simulink model "Project_microgrid__2016a"  (R2016a)
settings: Solver=VariableStepAuto  SolverMode=SingleTasking  StartTime=0.0  StopTime=0.3  RelTol=1e-3
undefined symbols (not defined in the file): D1, D11, Delta, DiscIntNeverNeededParam, find_system, Hydride, Metal, Nickel
libraries: powerlib x77, powerlib_meascontrol x31, sps_avr x7, simulink_extras x4, simulink x3, electricdrivelib x1, spsDieselMotorModel x1, re_lib x1
(part 2 of 5)

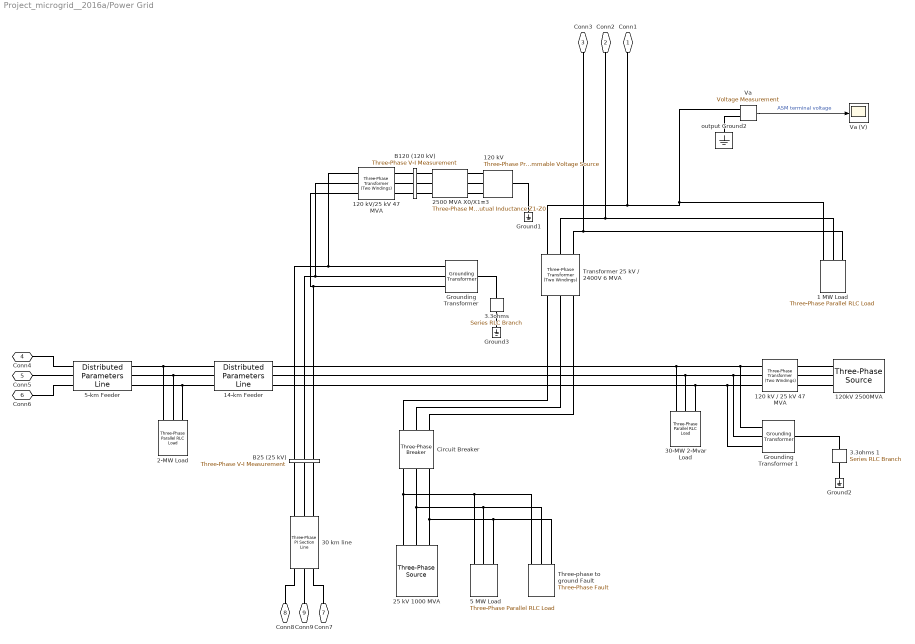
== system Project_microgrid__2016a/Power Grid ==
  1 MW Load : powerlib/Elements/Three-Phase Parallel RLC Load  LConnTagsString=A|B|C  Configuration=Y (grounded)  NominalVoltage=2400  Vabc=[1e3 1e3 1e3]  Vabcp=[1e3 1e3 1e3]  NominalFrequency=60  UnbalancedPower=off  ActivePower=1e+006  InductivePower=0  CapacitivePower=0  Pabc=[10e3 9e3 11e3]  QLabc=[100 90 110]  QCabc=[100 90 110]  Pabcp=[10e3 9e3 11e3]  QLabcp=[100 90 110]  QCabcp=[100 90 110]  Measurements=None  LoadType=constant Z
  120 kV : powerlib/Electrical Sources/Three-Phase Programmable Voltage Source  PositiveSequence=[120e3 0 60]  VariationEntity=Amplitude  VariationType=Table of time-amplitude pairs  VariationTypeAlt=Step  VariationStep=-0.2  VariationRate=10  VariationMagnitude=0.3  VariationFrequency=2  VariationTiming=[0.05 0.05+5/60]  VariationPhaseA=off  Amplitudes=[1 0.75 1.0]  TimeValues=[0 0.03 0.13]  HarmonicGeneration=off  HarmonicA=[1 -0.1 0 2]  HarmonicB=[2 0.15 35 2]*0  Timing="[0.1  2]"  BusType=swing  Pref=0  Qref=0  Qmin=-inf  Qmax=inf
  120 kV / 25 kV 47 MVA : powerlib/Elements/Three-Phase Transformer (Two Windings)  Winding1Connection=Yg  Winding2Connection=Delta (D1)  CoreType=Three single-phase transformers  SetSaturation=off  Hysteresis=off  DataFile='basic_model'  SetInitialFlux=off  Measurements=None  UNITS=pu  NominalPower=[47e6 50 ]  Winding1="[ 120e3  0.08/30   0.08 ]"  Winding2="[ 25e3  0.08/30  0.08]"  Rm=500  Lm=500  L0=0.5  Saturation="[ 0,0  ;  0.005,1.2  ;  1.0,1.4 ]"  InitialFluxes=[ 0.8 , -0.8 , 0.7 ]  BreakLoop=off  DiscreteSolver=Trapezoidal iterative  DataType=off  TransfoNumber=0
  120 kV/25 kV 47 MVA : powerlib/Elements/Three-Phase Transformer (Two Windings)  Winding1Connection=Yg  Winding2Connection=Delta (D1)  CoreType=Three single-phase transformers  SetSaturation=off  Hysteresis=off  DataFile='basic_model'  SetInitialFlux=off  Measurements=None  UNITS=pu  NominalPower=[47e6 60 ]  Winding1="[ 120e3  0.08/30   0.08 ]"  Winding2="[ 25e3  0.08/30  0.08]"  Rm=500  Lm=500  L0=0.5  Saturation="[ 0,0  ;  0.005,1.2  ;  1.0,1.4 ]"  InitialFluxes=[ 0.8 , -0.8 , 0.7 ]  BreakLoop=off  DiscreteSolver=Trapezoidal iterative  DataType=off  TransfoNumber=0
  120kV 2500MVA : powerlib/Electrical Sources/Three-Phase Source  InternalConnection=Yg  VoltagePhases=off  Voltage=150e3  PhaseAngle=0  Voltage_phases=[25e3 25e3 25e3]/sqrt(3)  PhaseAngles_phases=[0 -120 +120]  Frequency=50  NonIdealSource=on  SpecifyImpedance=on  Resistance=0.8929  Inductance=16.58e-3  ShortCircuitLevel=2500e6  BaseVoltage=120e3  XRratio=7  BusType=swing  Pref=0  Qref=0  Prefabc=[10e3, 10e3, 10e3]  Qrefabc=[0, 0, 0]  Qmin=-inf  Qmax=inf
  14-km Feeder : powerlib/Elements/Distributed Parameters Line  Phases=3  Frequency=50  Resistance=[0.1153 0.413]  Inductance=[1.05e-3 3.32e-3]  Capacitance=[11.33e-009 5.01e-009]  Length=14  x1=[-6e-05 5.24389383888345e-09 0 0;-5.6e-05 5.24712174909757e-09 0 0;-5.2e-05 5.25034137339023e-09 -4592.41120839546 -30084.6016905143;-4.8e-05 5.25355270667721e-09 -4554.60216686054 -30090.348929275;-4.4e-05 5.25675574388738e-09 -4516.7859329871 -30096.0486512675;-4e-05 5.2599504799627e-09 -4478.96256649216 -30101.7008474912;-3.6e-05 5.26313690985824e-09 -4441.13212710396 -30107.3055090205;-3.2e-05 5.26631502854221e-09 -4403.29467456193 -30112.8626270048;-2.8e-05 5.26948483099591e-09 -4365.45026861658 -30118.3721926688;-2.4e-05 5.27264631221381e-09 -4327.59896902939 -30123.834197312;-2e-05 5.27579946720347e-09 -4289.74083557272 -30129.2486323092;-1.6e-05 5.27894429098565e-09 -4251.87592802974 -30134.6154891103;-1.2e-05 5.28208077859424e-09 -4214.0043061943 -30139.9347592403;-8e-06 5.28520892507629e-09 -4176.12602987087 -30145.2064342993;-4e-06 5.28832872549204e-09 -4138.24115887441 -30150.4305059626]  x2=[-6e-05 5.41313383180429e-09 0 0;-5.6e-05 5.41611613444594e-09 0 0;-5.2e-05 5.41908988430093e-09 -4166.95541576399 -30299.6062453431;-4.8e-05 5.4220550766733e-09 -4128.87652753458 -30304.8186709667;-4.4e-05 5.42501170688062e-09 -4090.79111924556 -30309.9832411452;-4e-05 5.42795977025396e-09 -4052.69925103899 -30315.0999477229;-3.6e-05 5.43089926213792e-09 -4014.60098306712 -30320.1687826199;-3.2e-05 5.43383017789066e-09 -3976.49637549232 -30325.1897378317;-2.8e-05 5.43675251288384e-09 -3938.38548848696 -30330.1628054297;-2.4e-05 5.43966626250271e-09 -3900.26838223334 -30335.0879775607;-2e-05 5.44257142214605e-09 -3862.14511692358 -30339.9652464471;-1.6e-05 5.44546798722623e-09 -3824.01575275951 -30344.7946043871;-1.2e-05 5.44835595316917e-09 -3785.88034995259 -30349.5760437545;-8e-06 5.45123531541438e-09 -3747.73896872385 -30354.3095569987;-4e-06 5.45410606941495e-09 -3709.59166930372 -30358.9951366449]  x3=[-6e-05 2.19439041380111e-11 0 0;-5.6e-05 2.1954853930582e-11 0 0;-5.2e-05 2.19657690534419e-11 -28.5335833203508 -194.664312913599;-4.8e-05 2.19766494893542e-11 -28.2889384653752 -194.700015561698;-4.4e-05 2.19874952211371e-11 -28.0442489383045 -194.735410751896;-4e-05 2.1998306231664e-11 -27.7995151255367 -194.770498428299;-3.6e-05 2.20090825038626e-11 -27.55473741354 -194.8052785355;-3.2e-05 2.20198240207157e-11 -27.3099161888519 -194.839751018577;-2.8e-05 2.20305307652612e-11 -27.0650518380783 -194.873915823091;-2.4e-05 2.20412027205914e-11 -26.8201447478936 -194.907772895093;-2e-05 2.2051839869854e-11 -26.5751953050395 -194.941322181117;-1.6e-05 2.20624421962515e-11 -26.3302038963246 -194.974563628185;-1.2e-05 2.20730096830412e-11 -26.0851709086238 -195.007497183803;-8e-06 2.20835423135359e-11 -25.8400967288776 -195.040122795965;-4e-06 2.20940400711028e-11 -25.5949817440916 -195.072440413152]  x4=[-6e-05 -8.98993550684834e-12 0 0;-5.6e-05 -8.99242296522254e-12 0 0;-5.2e-05 -8.99489622333346e-12 -1.62633633076446 -2.68614935355567;-4.8e-05 -8.99735527727546e-12 -1.62295953271912 -2.6881909466271;-4.4e-05 -8.99980012316538e-12 -1.61958017179915 -2.69022829467809;-4e-05 -9.00223075714246e-12 -1.61619825334102 -2.6922613944914;-3.6e-05 -9.0046471753684e-12 -1.61281378268524 -2.69429024285649;-3.2e-05 -9.00704937402735e-12 -1.60942676517636 -2.69631483656952;-2.8e-05 -9.00943734932591e-12 -1.60603720616294 -2.69833517243338;-2.4e-05 -9.01181109749315e-12 -1.60264511099754 -2.7003512472577;-2e-05 -9.01417061478057e-12 -1.59925048503676 -2.70236305785881;-1.6e-05 -9.0165158974622e-12 -1.59585333364118 -2.70437060105978;-1.2e-05 -9.0188469418345e-12 -1.59245366217535 -2.70637387369045;-8e-06 -9.02116374421644e-12 -1.58905147600782 -2.70837287258735;-4e-06 -9.02346630094948e-12 -1.58564678051112 -2.71036759459381]  x5=5.70973484498186e-05  V1=ones(3,3)  V2=ones(3,3)  I1=ones(3,3)  I2=ones(3,3)  nHarmo=1  Measurements=None
  2-MW Load : powerlib/Elements/Three-Phase Parallel RLC Load  LConnTagsString=A|B|C  Configuration=Y (grounded)  NominalVoltage=25e3  Vabc=[1e3 1e3 1e3]  Vabcp=[1e3 1e3 1e3]  NominalFrequency=50  UnbalancedPower=off  ActivePower=2e6  InductivePower=0  CapacitivePower=0  Pabc=[10e3 9e3 11e3]  QLabc=[100 90 110]  QCabc=[100 90 110]  Pabcp=[10e3 9e3 11e3]  QLabcp=[100 90 110]  QCabcp=[100 90 110]  Measurements=None  LoadType=constant Z
  25 kV 1000 MVA : powerlib/Electrical Sources/Three-Phase Source  InternalConnection=Yg  VoltagePhases=off  Voltage=(25000)*1  PhaseAngle=2.1395e-05  Voltage_phases=[25e3 25e3 25e3]/sqrt(3)  PhaseAngles_phases=[0 -120 +120]  Frequency=60  NonIdealSource=on  SpecifyImpedance=on  Resistance=25^2/1000/10  Inductance=25^2/1000/377  ShortCircuitLevel=1000e6  BaseVoltage=25e3  XRratio=10  BusType=swing  Pref=0  Qref=0  Prefabc=[10e3, 10e3, 10e3]  Qrefabc=[0, 0, 0]  Qmin=-Inf  Qmax=Inf
  2500 MVA X0/X1=3 : powerlib/Elements/Three-Phase Mutual Inductance Z1-Z0  LConnTagsString=a|b|c  RConnTagsString=A|B|C  PositiveSequence="[0.1  1.0/(2*pi*60)] *120e3^2/2500e6"  ZeroSequence="[0.3  3.0/(2*pi*60)] *120e3^2/2500e6"
  "3.3ohms " : powerlib/Elements/Series RLC Branch  LConnTagsString=__new0  RConnTagsString=__new0  BranchType=R  Resistance=3.3  Inductance=[]  SetiL0=off  InitialCurrent=0  Capacitance=[]  Setx0=off  InitialVoltage=0  Measurements=None
  3.3ohms 1 : powerlib/Elements/Series RLC Branch  LConnTagsString=__new0  RConnTagsString=__new0  BranchType=R  Resistance=3.3  Inductance=[]  SetiL0=off  InitialCurrent=0  Capacitance=[]  Setx0=off  InitialVoltage=0  Measurements=None
  30 km line : powerlib/Elements/Three-Phase PI Section Line  LConnTagsString=a|b|c  RConnTagsString=A|B|C  Frequency=60  Resistances=[0.1153 0.413]  Inductances=[1.05e-3 3.32e-3]  Capacitances=[11.33e-009 5.01e-009]  Length=30
  30-MW 2-Mvar Load : powerlib/Elements/Three-Phase Parallel RLC Load  LConnTagsString=A|B|C  Configuration=Y (grounded)  NominalVoltage=25e3  Vabc=[1e3 1e3 1e3]  Vabcp=[1e3 1e3 1e3]  NominalFrequency=50  UnbalancedPower=off  ActivePower=30e6  InductivePower=2e6  CapacitivePower=0  Pabc=[10e3 9e3 11e3]  QLabc=[100 90 110]  QCabc=[100 90 110]  Pabcp=[10e3 9e3 11e3]  QLabcp=[100 90 110]  QCabcp=[100 90 110]  Measurements=None  LoadType=constant Z
  5 MW Load : powerlib/Elements/Three-Phase Parallel RLC Load  LConnTagsString=A|B|C  Configuration=Y (grounded)  NominalVoltage=25e3  Vabc=[1e3 1e3 1e3]  Vabcp=[1e3 1e3 1e3]  NominalFrequency=60  UnbalancedPower=off  ActivePower=5e+006  InductivePower=0  CapacitivePower=0  Pabc=[10e3 9e3 11e3]  QLabc=[100 90 110]  QCabc=[100 90 110]  Pabcp=[10e3 9e3 11e3]  QLabcp=[100 90 110]  QCabcp=[100 90 110]  Measurements=None  LoadType=constant Z
  5-km Feeder : powerlib/Elements/Distributed Parameters Line  Phases=3  Frequency=50  Resistance=[0.1153 0.413]  Inductance=[1.05e-3 3.32e-3]  Capacitance=[11.33e-009 5.01e-009]  Length=5  x1=[-2.4e-05 5.33826007366157e-09 -4328.38679732203 -30125.1982220609;-2e-05 5.34139179699889e-09 -4290.52694915972 -30130.6136459951;-1.6e-05 5.34451508554948e-09 -4252.66032566971 -30135.9814895777;-1.2e-05 5.34762993438124e-09 -4214.78698664858 -30141.301744332;-8e-06 5.35073633857541e-09 -4176.90699190349 -30146.5744018567;-4e-06 5.35383429322654e-09 -4139.02040125213 -30151.7994538255]  x2=[-2.4e-05 5.27264631221381e-09 -4327.59896902939 -30123.834197312;-2e-05 5.27579946720347e-09 -4289.74083557272 -30129.2486323092;-1.6e-05 5.27894429098565e-09 -4251.87592802974 -30134.6154891103;-1.2e-05 5.28208077859424e-09 -4214.0043061943 -30139.9347592403;-8e-06 5.28520892507629e-09 -4176.12602987087 -30145.2064342993;-4e-06 5.28832872549204e-09 -4138.24115887441 -30150.4305059626]  x3=[-2.4e-05 2.33940631713485e-13 -13.5809735435642 -98.9468276004231;-2e-05 2.2688527897437e-13 -13.4566226025095 -98.9638158253433;-1.6e-05 2.19829567952431e-13 -13.332250411611 -98.9806477728902;-1.2e-05 2.12773509789599e-13 -13.2078571672692 -98.9973234164837;-8e-06 2.05717115628352e-13 -13.0834430659182 -99.0138427297907;-4e-06 1.98660396611699e-13 -12.9590083040247 -99.030205686725]  x4=[-2.4e-05 1.33449662502356e-11 -15.3482236981344 -98.6065510111038;-2e-05 1.33597788176704e-11 -15.2242989657759 -98.6257602961521;-1.6e-05 1.33745702881909e-11 -15.1003501921712 -98.6448138376629;-1.2e-05 1.33893406384393e-11 -14.9763775730525 -98.6637116055479;-8e-06 1.34040898450913e-11 -14.8523813041894 -98.6824535699651;-4e-06 1.34188178848558e-11 -14.7283615813888 -98.7010397013183]  x5=2.03919101606495e-05  V1=ones(3,3)  V2=ones(3,3)  I1=ones(3,3)  I2=ones(3,3)  nHarmo=1  Measurements=None
  B120 (120 kV) : powerlib/Measurements/Three-Phase V-I Measurement  VoltageMeasurement=no  SetLabelV=off  LabelV=Vabc_B120  Vpu=off  VpuLL=off  CurrentMeasurement=no  SetLabelI=on  LabelI=Iabc_B120  Ipu=off  Pbase=100e6  Vbase=120e3  OutputType=Complex  PhasorSimulation=off  PSBequivalent=0
  B25 (25 kV) : powerlib/Measurements/Three-Phase V-I Measurement  VoltageMeasurement=phase-to-ground  SetLabelV=on  LabelV=Vabc_B25  Vpu=off  VpuLL=off  CurrentMeasurement=yes  SetLabelI=on  LabelI=Iabc_B25  Ipu=off  Pbase=10e6  Vbase=25e3  OutputType=Complex  PhasorSimulation=off  PSBequivalent=0
  Circuit Breaker : powerlib/Elements/Three-Phase Breaker  InitialState=closed  SwitchA=on  SwitchB=on  SwitchC=on  SwitchTimes=[0.2]  External=off  BreakerResistance=0.01  SnubberResistance=1e5  SnubberCapacitance=inf  Measurements=None
      settings: AttributesFormatString=\n
  Ground1 : powerlib/Elements/Ground  LConnTagsString=a
  Ground2 : powerlib/Elements/Ground  LConnTagsString=a
  Ground3 : powerlib/Elements/Ground  LConnTagsString=a
  "Grounding Transformer " : powerlib/Elements/Grounding Transformer   UNITS=pu  NominalPower="[100e6   60]"  NominalVoltage=25e3  ZeroSequenceImpedance_pu=[0.025 0.75]  MagnetizationBranch_pu=[500 500]  ZeroSequenceImpedance_SI=[0.052083 589.05]  MagnetizationBranch_SI=[1041.7 3.927e+005]  Measurements=None
  Grounding Transformer 1 : powerlib/Elements/Grounding Transformer   UNITS=pu  NominalPower="[150e6   50]"  NominalVoltage=25e3  ZeroSequenceImpedance_pu=[0.025 0.75]  MagnetizationBranch_pu=[500 500]  ZeroSequenceImpedance_SI=[0.052083 589.05]  MagnetizationBranch_SI=[1041.7 3.927e+005]  Measurements=None
  Three-phase to ground Fault : powerlib/Elements/Three-Phase Fault  InitialStates=0  FaultA=on  FaultB=on  FaultC=on  GroundFault=on  SwitchTimes=[ 0.1 0.4]  External=off  SwitchStatus=NaN  FaultResistance=0.01  GroundResistance=0.001  SnubberResistance=inf  SnubberCapacitance=inf  Measurements=None
  Transformer 25 kV / 2400V 6 MVA : powerlib/Elements/Three-Phase Transformer (Two Windings)  Winding1Connection=Yg  Winding2Connection=Delta (D1)  CoreType=Three single-phase transformers  SetSaturation=off  Hysteresis=off  DataFile='hysteresis'  SetInitialFlux=off  Measurements=None  UNITS=pu  NominalPower=[ 6e6 , 60 ]  Winding1=[ 25e3 , 0.0015 , 0.03]  Winding2=[ 2.4e3 , 0.0015 , 0.03 ]  Rm=200  Lm=200  L0=0.5  Saturation="[ 0,0  ;  0.005,1.2  ;  1.0,1.4 ]"  InitialFluxes=[ 0.8 , -0.8 , 0.7 ]  BreakLoop=off  DiscreteSolver=Trapezoidal iterative  DataType=off  TransfoNumber=0
  Va : powerlib/Measurements/Voltage Measurement  Tag=PoWeRsYsTeMmEaSuReMeNt  PhasorSimulation=off  OutputType=Magnitude  PSBequivalent=0
  Va (V) : Scope
  output Ground2 : powerlib/Elements/Ground  LConnTagsString=a
  Conn1 : PMIOPort  Side=Left
  Conn2 : PMIOPort  Port=2  Side=Left
  Conn3 : PMIOPort  Port=3  Side=Left
  Conn4 : PMIOPort  Port=4  Side=Left
  Conn5 : PMIOPort  Port=5  Side=Left
  Conn6 : PMIOPort  Port=6  Side=Left
  Conn7 : PMIOPort  Port=7  Side=Left
  Conn8 : PMIOPort  Port=8  Side=Left
  Conn9 : PMIOPort  Port=9  Side=Left
  wires:
  Va/1 -> Va (V)/1  "ASM terminal voltage"
  connections:
  B120 (120 kV)/RConn1 -- 120 kV/25 kV 47 MVA/LConn1
  "3.3ohms "/RConn1 -- Ground3/LConn1
  Circuit Breaker/LConn1 -- 25 kV 1000 MVA/RConn1 -- 5 MW Load/LConn1 -- Three-phase to ground Fault/LConn1
  "Grounding Transformer "/LConn3 -- 120 kV/25 kV 47 MVA/RConn3 -- B25 (25 kV)/LConn3
  B120 (120 kV)/RConn3 -- 120 kV/25 kV 47 MVA/LConn3
  25 kV 1000 MVA/RConn3 -- Circuit Breaker/LConn3 -- 5 MW Load/LConn3 -- Three-phase to ground Fault/LConn3
  Conn6/RConn1 -- 5-km Feeder/LConn3
  Transformer 25 kV / 2400V 6 MVA/RConn3 -- Conn3/RConn1 -- 1 MW Load/LConn3
  2-MW Load/LConn3 -- 5-km Feeder/RConn3 -- 14-km Feeder/LConn3
  B120 (120 kV)/LConn3 -- 2500 MVA X0/X1=3/RConn3
  "3.3ohms "/LConn1 -- "Grounding Transformer "/RConn1
  120 kV/RConn1 -- 2500 MVA X0/X1=3/LConn1
  120 kV / 25 kV 47 MVA/LConn1 -- 120kV 2500MVA/RConn1
  120 kV / 25 kV 47 MVA/LConn2 -- 120kV 2500MVA/RConn2
  B25 (25 kV)/RConn3 -- 30 km line/LConn3
  B120 (120 kV)/LConn2 -- 2500 MVA X0/X1=3/RConn2
  2-MW Load/LConn2 -- 5-km Feeder/RConn2 -- 14-km Feeder/LConn2
  Transformer 25 kV / 2400V 6 MVA/RConn2 -- Conn2/RConn1 -- 1 MW Load/LConn2
  120 kV/RConn3 -- 2500 MVA X0/X1=3/LConn3
  30-MW 2-Mvar Load/LConn3 -- 14-km Feeder/RConn3 -- 120 kV / 25 kV 47 MVA/RConn3 -- Grounding Transformer 1/LConn3
  B25 (25 kV)/LConn2 -- "Grounding Transformer "/LConn2 -- 120 kV/25 kV 47 MVA/RConn2
  B120 (120 kV)/LConn1 -- 2500 MVA X0/X1=3/RConn1
  Grounding Transformer 1/RConn1 -- 3.3ohms 1/LConn1
  B25 (25 kV)/RConn1 -- 30 km line/LConn1
  120 kV/RConn2 -- 2500 MVA X0/X1=3/LConn2
  Conn9/RConn1 -- 30 km line/RConn2
  120 kV / 25 kV 47 MVA/LConn3 -- 120kV 2500MVA/RConn3
  Ground1/LConn1 -- 120 kV/LConn1
  B25 (25 kV)/RConn2 -- 30 km line/LConn2
  2-MW Load/LConn1 -- 5-km Feeder/RConn1 -- 14-km Feeder/LConn1
  30-MW 2-Mvar Load/LConn1 -- 120 kV / 25 kV 47 MVA/RConn1 -- Grounding Transformer 1/LConn1 -- 14-km Feeder/RConn1
  30-MW 2-Mvar Load/LConn2 -- 120 kV / 25 kV 47 MVA/RConn2 -- Grounding Transformer 1/LConn2 -- 14-km Feeder/RConn2
  B25 (25 kV)/LConn1 -- "Grounding Transformer "/LConn1 -- 120 kV/25 kV 47 MVA/RConn1
  B120 (120 kV)/RConn2 -- 120 kV/25 kV 47 MVA/LConn2
  3.3ohms 1/RConn1 -- Ground2/LConn1
  1 MW Load/LConn1 -- Va/LConn1 -- Transformer 25 kV / 2400V 6 MVA/RConn1 -- Conn1/RConn1
  Circuit Breaker/RConn2 -- Transformer 25 kV / 2400V 6 MVA/LConn2
  output Ground2/LConn1 -- Va/LConn2
  Three-phase to ground Fault/LConn2 -- 25 kV 1000 MVA/RConn2 -- Circuit Breaker/LConn2 -- 5 MW Load/LConn2
  Circuit Breaker/RConn3 -- Transformer 25 kV / 2400V 6 MVA/LConn3
  Circuit Breaker/RConn1 -- Transformer 25 kV / 2400V 6 MVA/LConn1
  Conn8/RConn1 -- 30 km line/RConn1
  Conn4/RConn1 -- 5-km Feeder/LConn1
  Conn5/RConn1 -- 5-km Feeder/LConn2
  Conn7/RConn1 -- 30 km line/RConn3

== system Project_microgrid__2016a/Relay G ==
  AC Time Overcurrent Relay2 : Subsystem  mask(AC Time Overcurrent Relay Block){tcpopup=Definite Minimum Time, k=0, alpha=0.02, B=0, PS=100%, TMS=0.1, TDS=5, CTpri=300, CTsec=5, Freq=60, RMSInit=0}
      mask prompts: tcpopup "Trip Characteristic"; PS "Plug Setting (PS) / Low-set (I >)"; TMS "Time Multiplier Setting (TMS)"; TDS "Time Delay Setting (TDS) in sec"; CTpri "Current Transformer Primary (A)"; CTsec "Current Transformer Secondary (A)"; Freq "Fundamental frequency (Hz):"; RMSInit "Initial RMS value:"
      mask help:
      | AC Time Overcurrent Relay Block developed by Dr Rodney Tan
      | Version 1.0 (Jun 2016)
      |
      | AC Time Overcurrent Relay (ANSI/IEEE C37.2 device number 51) that operates when the current exceeds a predetermined value.
      |
      | This relay operates with either a Definite Minimum Time (DMT) or Inverse Definite Minimum Time (IDMT) characteristic.
      |
      | This relay support both IEC 60255 Standard and IEEE Standard C37.112-1996 IDMT trip characteristic.
      mask Help:
      | <b><u>Block Setting</u></b>
      | <b>Trip Characteristic</b>
      | Relay operation mode selection of Definite Minimum Time (DMT), IEC 60255 Standard or IEEE Standard C37.112-1996 Inverse Definite Minimum Time (IDMT).
      | 
      | <b>Plug-Setting(PS) / Low-set (I >)</b>
      | Specify relay pick-up current based on current transformer rating ranging from 25% to 200% with 25% step interval.
      | 
      | <b>Time Multiplier Setting (TMS)</b>
      | Specify time delay multiplier ranging from 0.05 to 1.0 for IDMT relay operation. This setting will be disabled DMT relay operation mode.
      | 
      | <b>Plot Curve Button</b>
      | Plot current Inverse Definite Minimum Time trip curve.
      | 
      | <b>Time Delay Setting (TDS)</b>
      | Specify time delay ranging from 0.05sec to 99sec for Definite Minimum Time relay operation. This setting will be disabled in IDMT relay operation mode.
      | 
      | <b>Current Transformer Primary (A)</b>
      | Specify current transformer primary in Ampere.
      | 
      | <b>Current Transformer Secondary (A)</b>
      | Specify current transformer secondary in Ampere.
      | 
      | <b>Fundamental Frequency (Hz)</b>
      | Specify the RMS current measurement fundamental frequency, in hertz, of the input signal.
      | 
      | <b>Initial RMS Value</b>
      | Specify the RMS current measurement initial RMS value of the output signal.
      | 
      | <b><u>Block Input Output</u></b>
      | <b>I</b>
      | Current input to the AC time overcurrent relay
      | 
      | <b>trip</b>
      | Trip control signal output (1-0), commonly connected to circuit breaker
      | 
      | <b>OT</b>
      | Relay operating time output
      mask TypeOptions tcpopup: Definite Minimum Time | IEC Standard Inverse | IEC Very Inverse | IEC Long Time Inverse | IEC Extremely Inverse | IEC Ultra Inverse | IEEE Moderately Inverse | IEEE Very Inverse | IEEE Extremely Inverse
      mask Callback tcpopup:
      | switch(get_param(gcb,'tcpopup'))
      |     case 'IEC Standard Inverse'
      |         set_param(gcb,'k','0.14');
      |         set_param(gcb,'alpha','0.02');
      |         set_param(gcb,'B','0');
      |         set_param(gcb,'MaskEnables',{'on','off','off','off',...
      |                   'on','on','off','on','on','on','on'});
      |     case 'IEC Very Inverse'
      |         set_param(gcb,'k','13.5');
      |         set_param(gcb,'alpha','1');
      |         set_param(gcb,'B','0');
      |         set_param(gcb,'MaskEnables',{'on','off','off','off',...
      |                   'on','on','off','on','on','on','on'});
      |     case 'IEC Long Time Inverse'
      |         set_param(gcb,'k','120');
      |         set_param(gcb,'alpha','1');
      |         set_param(gcb,'B','0');
      |         set_param(gcb,'MaskEnables',{'on','off','off','off',...
      |                   'on','on','off','on','on','on','on'});
      |     case 'IEC Extremely Inverse'
      |         set_param(gcb,'k','80');
      |         set_param(gcb,'alpha','2');
      |         set_param(gcb,'B','0');
      |         set_param(gcb,'MaskEnables',{'on','off','off','off',...
      |                   'on','on','off','on','on','on','on'});
      |     case 'IEC Ultra Inverse'
      |         set_param(gcb,'k','315.2');
      |         set_param(gcb,'alpha','2.5');
      |         set_param(gcb,'B','0');
      |         set_param(gcb,'MaskEnables',{'on','off','off','off',...
      |                   'on','on','off','on','on','on','on'});
      |     case 'IEEE Moderately Inverse'
      |         set_param(gcb,'k','0.0515');
      |         set_param(gcb,'alpha','0.02');
      |         set_param(gcb,'B','0.114');
      |         set_param(gcb,'MaskEnables',{'on','off','off','off',...
      |                   'on','on','off','on','on','on','on'});
      |     case 'IEEE Very Inverse'
      |         set_param(gcb,'k','19.61');
      |         set_param(gcb,'alpha','2');
      |         set_param(gcb,'B','0.491');
      |         set_param(gcb,'MaskEnables',{'on','off','off','off',...
      |                   'on','on','off','on','on','on','on'});
      |     case 'IEEE Extremely Inverse'
      |         set_param(gcb,'k','28.2');
      |         set_param(gcb,'alpha','2');
      |         set_param(gcb,'B','0.1217');
      |         set_param(gcb,'MaskEnables',{'on','off','off','off',...
      |                   'on','on','off','on','on','on','on'});
      |     otherwise
      |         set_param(gcb,'k','0');
      |         set_param(gcb,'MaskEnables',{'on','off','off','off',...
      |                   'on','off','on','on','on','on','on'});
      | end
      mask TypeOptions PS: 25% | 50% | 75% | 100% | 125% | 150% | 175% | 200%
      mask TypeOptions TMS: 0.05 | 0.1 | 0.15 | 0.2 | 0.25 | 0.3 | 0.35 | 0.4 | 0.45 | 0.5 | 0.55 | 0.6 | 0.65 | 0.7 | 0.75 | 0.8 | 0.85 | 0.9 | 0.95 | 1.0
      mask Callback TDS:
      | TDS = str2double(get_param(gcb,'TDS'));
      | if (TDS > 99)||(TDS < 0.05)||isnan(TDS)
      |     msgbox('TDS must be in the range of 0.05-99 sec',...
      |     'Invalid Value !','error');
      |     set_param(gcb,'TDS','0.1');
      | end
      mask TypeOptions Freq: Irms/Freq
      mask TypeOptions RMSInit: Irms/RMSInit
      mask DialogControl plotbutton Prompt: Plot Curve
      mask DialogControl plotbutton Callback:
      | % Plotting IDMT Curve
      | TMS = str2num(get_param(gcb,'TMS'));
      | k = str2num(get_param(gcb,'k'));
      | alpha = str2num(get_param(gcb,'alpha'));
      | B = str2num(get_param(gcb,'B'));
      | I = 1:20;
      | td = ((k./((I.^alpha)-1))+B)*TMS;
      | loglog(td);
      | set(gcf, 'Position', [200 150 300 500]);
      | switch(get_param(gcb,'tcpopup'))
      |     case 'IEC Standard Inverse'
      |         title('IEC Standard Inverse');
      |         set(gca, 'YTick', (1:10));
      |         ylim([0.1 10]);
      |     case 'IEC Very Inverse'
      |         title('IEC Very Inverse');
      |         set(gca, 'YTick', (1:2:15));
      |         ylim([0.01 15]);
      |     case 'IEC Long Time Inverse'
      |         title('IEC Long Time Inverse');
      |         set(gca, 'YTick', (0:20:120));
      |         ylim([0.1 120]);
      |     case 'IEC Extremely Inverse'
      |         title('IEC Extremely Inverse');
      |         set(gca, 'YTick', (0:5:30));
      |         ylim([0.01 30]);
      |     case 'IEC Ultra Inverse'
      |         title('IEC Ultra Inverse');
      |         set(gca, 'YTick', (0:20:100));
      |         ylim([0.01 100]);
      |     case 'IEEE Moderately Inverse'
      |         title('IEEE Moderately Inverse');
      |         set(gca, 'YTick', (1:5));
      |         ylim([0.01 5]);
      |     case 'IEEE Very Inverse'
      |         title('IEEE Very Inverse');
      |         set(gca, 'YTick', (1:10));
      |         ylim([0.01 10]);
      |     case 'IEEE Extremely Inverse'
      |         title('IEEE Extremely Inverse');
      |         set(gca, 'YTick', (1:10));
      |         ylim([0.01 10]);
      | end
      | 
      | set(gca, 'XTick', [1:10 20]);
      | xlim([1 30]);
      | xlabel('Current (Multiples of Plug Setting)');
      | ylabel('Operating Time (sec)');
      | grid on;
      mask DialogControl RMS Prompt: RMS Current Measurement
      mask Display:
      | disp('(51)');
      | port_label('input', 1, 'I');
      | port_label('output', 1, 'trip');
      | port_label('output', 2, 'OT');
  Display : Display
  Output1 : Subsystem
  Three-Phase V-I Measurement : powerlib/Measurements/Three-Phase V-I Measurement  VoltageMeasurement=no  SetLabelV=off  LabelV=Vabc  Vpu=off  VpuLL=off  CurrentMeasurement=yes  SetLabelI=off  LabelI=Iabc  Ipu=off  Pbase=100e6  Vbase=500e3  OutputType=Complex  PhasorSimulation=off  PSBequivalent=0
  Three-Phase Breaker : powerlib/Elements/Three-Phase Breaker  InitialState=closed  SwitchA=on  SwitchB=on  SwitchC=on  SwitchTimes="[1/60  5/60]"  External=on  BreakerResistance=0.001  SnubberResistance=1e6  SnubberCapacitance=inf  Measurements=None
  A : PMIOPort  Side=Left
  a : PMIOPort  Port=2  Side=Right
  B : PMIOPort  Port=3  Side=Left
  b : PMIOPort  Port=4  Side=Right
  C : PMIOPort  Port=5  Side=Left
  c : PMIOPort  Port=6  Side=Right
  wires:
  Three-Phase V-I Measurement/1 -> Output1/1(Signal), AC Time Overcurrent Relay2/1(I)  "Iabc"
  AC Time Overcurrent Relay2/2(OT) -> Display/1
  AC Time Overcurrent Relay2/1(C.B) -> Three-Phase Breaker/1  "Relay C"
  connections:
  Three-Phase Breaker/RConn2 -- Three-Phase V-I Measurement/LConn2
  Three-Phase V-I Measurement/RConn2 -- b/RConn1
  Three-Phase V-I Measurement/LConn1 -- Three-Phase Breaker/RConn1
  Three-Phase Breaker/LConn2 -- B/RConn1
  Three-Phase V-I Measurement/RConn1 -- a/RConn1
  Three-Phase Breaker/RConn3 -- Three-Phase V-I Measurement/LConn3
  Three-Phase Breaker/LConn3 -- C/RConn1
  Three-Phase V-I Measurement/RConn3 -- c/RConn1
  Three-Phase Breaker/LConn1 -- A/RConn1

== system Project_microgrid__2016a/Relay PV ==
  AC Time Overcurrent Relay2 : Subsystem  mask(AC Time Overcurrent Relay Block){tcpopup=Definite Minimum Time, k=0, alpha=0.02, B=0, PS=100%, TMS=0.1, TDS=5, CTpri=300, CTsec=5, Freq=60, RMSInit=0}
      mask prompts: tcpopup "Trip Characteristic"; PS "Plug Setting (PS) / Low-set (I >)"; TMS "Time Multiplier Setting (TMS)"; TDS "Time Delay Setting (TDS) in sec"; CTpri "Current Transformer Primary (A)"; CTsec "Current Transformer Secondary (A)"; Freq "Fundamental frequency (Hz):"; RMSInit "Initial RMS value:"
      mask help:
      | AC Time Overcurrent Relay Block developed by Dr Rodney Tan
      | Version 1.0 (Jun 2016)
      |
      | AC Time Overcurrent Relay (ANSI/IEEE C37.2 device number 51) that operates when the current exceeds a predetermined value.
      |
      | This relay operates with either a Definite Minimum Time (DMT) or Inverse Definite Minimum Time (IDMT) characteristic.
      |
      | This relay support both IEC 60255 Standard and IEEE Standard C37.112-1996 IDMT trip characteristic.
      mask Help:
      | <b><u>Block Setting</u></b>
      | <b>Trip Characteristic</b>
      | Relay operation mode selection of Definite Minimum Time (DMT), IEC 60255 Standard or IEEE Standard C37.112-1996 Inverse Definite Minimum Time (IDMT).
      | 
      | <b>Plug-Setting(PS) / Low-set (I >)</b>
      | Specify relay pick-up current based on current transformer rating ranging from 25% to 200% with 25% step interval.
      | 
      | <b>Time Multiplier Setting (TMS)</b>
      | Specify time delay multiplier ranging from 0.05 to 1.0 for IDMT relay operation. This setting will be disabled DMT relay operation mode.
      | 
      | <b>Plot Curve Button</b>
      | Plot current Inverse Definite Minimum Time trip curve.
      | 
      | <b>Time Delay Setting (TDS)</b>
      | Specify time delay ranging from 0.05sec to 99sec for Definite Minimum Time relay operation. This setting will be disabled in IDMT relay operation mode.
      | 
      | <b>Current Transformer Primary (A)</b>
      | Specify current transformer primary in Ampere.
      | 
      | <b>Current Transformer Secondary (A)</b>
      | Specify current transformer secondary in Ampere.
      | 
      | <b>Fundamental Frequency (Hz)</b>
      | Specify the RMS current measurement fundamental frequency, in hertz, of the input signal.
      | 
      | <b>Initial RMS Value</b>
      | Specify the RMS current measurement initial RMS value of the output signal.
      | 
      | <b><u>Block Input Output</u></b>
      | <b>I</b>
      | Current input to the AC time overcurrent relay
      | 
      | <b>trip</b>
      | Trip control signal output (1-0), commonly connected to circuit breaker
      | 
      | <b>OT</b>
      | Relay operating time output
      mask TypeOptions tcpopup: Definite Minimum Time | IEC Standard Inverse | IEC Very Inverse | IEC Long Time Inverse | IEC Extremely Inverse | IEC Ultra Inverse | IEEE Moderately Inverse | IEEE Very Inverse | IEEE Extremely Inverse
      mask Callback tcpopup:
      | switch(get_param(gcb,'tcpopup'))
      |     case 'IEC Standard Inverse'
      |         set_param(gcb,'k','0.14');
      |         set_param(gcb,'alpha','0.02');
      |         set_param(gcb,'B','0');
      |         set_param(gcb,'MaskEnables',{'on','off','off','off',...
      |                   'on','on','off','on','on','on','on'});
      |     case 'IEC Very Inverse'
      |         set_param(gcb,'k','13.5');
      |         set_param(gcb,'alpha','1');
      |         set_param(gcb,'B','0');
      |         set_param(gcb,'MaskEnables',{'on','off','off','off',...
      |                   'on','on','off','on','on','on','on'});
      |     case 'IEC Long Time Inverse'
      |         set_param(gcb,'k','120');
      |         set_param(gcb,'alpha','1');
      |         set_param(gcb,'B','0');
      |         set_param(gcb,'MaskEnables',{'on','off','off','off',...
      |                   'on','on','off','on','on','on','on'});
      |     case 'IEC Extremely Inverse'
      |         set_param(gcb,'k','80');
      |         set_param(gcb,'alpha','2');
      |         set_param(gcb,'B','0');
      |         set_param(gcb,'MaskEnables',{'on','off','off','off',...
      |                   'on','on','off','on','on','on','on'});
      |     case 'IEC Ultra Inverse'
      |         set_param(gcb,'k','315.2');
      |         set_param(gcb,'alpha','2.5');
      |         set_param(gcb,'B','0');
      |         set_param(gcb,'MaskEnables',{'on','off','off','off',...
      |                   'on','on','off','on','on','on','on'});
      |     case 'IEEE Moderately Inverse'
      |         set_param(gcb,'k','0.0515');
      |         set_param(gcb,'alpha','0.02');
      |         set_param(gcb,'B','0.114');
      |         set_param(gcb,'MaskEnables',{'on','off','off','off',...
      |                   'on','on','off','on','on','on','on'});
      |     case 'IEEE Very Inverse'
      |         set_param(gcb,'k','19.61');
      |         set_param(gcb,'alpha','2');
      |         set_param(gcb,'B','0.491');
      |         set_param(gcb,'MaskEnables',{'on','off','off','off',...
      |                   'on','on','off','on','on','on','on'});
      |     case 'IEEE Extremely Inverse'
      |         set_param(gcb,'k','28.2');
      |         set_param(gcb,'alpha','2');
      |         set_param(gcb,'B','0.1217');
      |         set_param(gcb,'MaskEnables',{'on','off','off','off',...
      |                   'on','on','off','on','on','on','on'});
      |     otherwise
      |         set_param(gcb,'k','0');
      |         set_param(gcb,'MaskEnables',{'on','off','off','off',...
      |                   'on','off','on','on','on','on','on'});
      | end
      mask TypeOptions PS: 25% | 50% | 75% | 100% | 125% | 150% | 175% | 200%
      mask TypeOptions TMS: 0.05 | 0.1 | 0.15 | 0.2 | 0.25 | 0.3 | 0.35 | 0.4 | 0.45 | 0.5 | 0.55 | 0.6 | 0.65 | 0.7 | 0.75 | 0.8 | 0.85 | 0.9 | 0.95 | 1.0
      mask Callback TDS:
      | TDS = str2double(get_param(gcb,'TDS'));
      | if (TDS > 99)||(TDS < 0.05)||isnan(TDS)
      |     msgbox('TDS must be in the range of 0.05-99 sec',...
      |     'Invalid Value !','error');
      |     set_param(gcb,'TDS','0.1');
      | end
      mask TypeOptions Freq: Irms/Freq
      mask TypeOptions RMSInit: Irms/RMSInit
      mask DialogControl plotbutton Prompt: Plot Curve
      mask DialogControl plotbutton Callback:
      | % Plotting IDMT Curve
      | TMS = str2num(get_param(gcb,'TMS'));
      | k = str2num(get_param(gcb,'k'));
      | alpha = str2num(get_param(gcb,'alpha'));
      | B = str2num(get_param(gcb,'B'));
      | I = 1:20;
      | td = ((k./((I.^alpha)-1))+B)*TMS;
      | loglog(td);
      | set(gcf, 'Position', [200 150 300 500]);
      | switch(get_param(gcb,'tcpopup'))
      |     case 'IEC Standard Inverse'
      |         title('IEC Standard Inverse');
      |         set(gca, 'YTick', (1:10));
      |         ylim([0.1 10]);
      |     case 'IEC Very Inverse'
      |         title('IEC Very Inverse');
      |         set(gca, 'YTick', (1:2:15));
      |         ylim([0.01 15]);
      |     case 'IEC Long Time Inverse'
      |         title('IEC Long Time Inverse');
      |         set(gca, 'YTick', (0:20:120));
      |         ylim([0.1 120]);
      |     case 'IEC Extremely Inverse'
      |         title('IEC Extremely Inverse');
      |         set(gca, 'YTick', (0:5:30));
      |         ylim([0.01 30]);
      |     case 'IEC Ultra Inverse'
      |         title('IEC Ultra Inverse');
      |         set(gca, 'YTick', (0:20:100));
      |         ylim([0.01 100]);
      |     case 'IEEE Moderately Inverse'
      |         title('IEEE Moderately Inverse');
      |         set(gca, 'YTick', (1:5));
      |         ylim([0.01 5]);
      |     case 'IEEE Very Inverse'
      |         title('IEEE Very Inverse');
      |         set(gca, 'YTick', (1:10));
      |         ylim([0.01 10]);
      |     case 'IEEE Extremely Inverse'
      |         title('IEEE Extremely Inverse');
      |         set(gca, 'YTick', (1:10));
      |         ylim([0.01 10]);
      | end
      | 
      | set(gca, 'XTick', [1:10 20]);
      | xlim([1 30]);
      | xlabel('Current (Multiples of Plug Setting)');
      | ylabel('Operating Time (sec)');
      | grid on;
      mask DialogControl RMS Prompt: RMS Current Measurement
      mask Display:
      | disp('(51)');
      | port_label('input', 1, 'I');
      | port_label('output', 1, 'trip');
      | port_label('output', 2, 'OT');
  Display : Display
  Three-Phase V-I Measurement : powerlib/Measurements/Three-Phase V-I Measurement  VoltageMeasurement=no  SetLabelV=off  LabelV=Vabc  Vpu=off  VpuLL=off  CurrentMeasurement=yes  SetLabelI=off  LabelI=Iabc  Ipu=off  Pbase=100e6  Vbase=500e3  OutputType=Complex  PhasorSimulation=off  PSBequivalent=0
  Three-Phase Breaker : powerlib/Elements/Three-Phase Breaker  InitialState=closed  SwitchA=on  SwitchB=on  SwitchC=on  SwitchTimes="[1/60  5/60]"  External=on  BreakerResistance=0.001  SnubberResistance=1e6  SnubberCapacitance=inf  Measurements=None
  A : PMIOPort  Side=Left
  a : PMIOPort  Port=2  Side=Right
  B : PMIOPort  Port=3  Side=Left
  b : PMIOPort  Port=4  Side=Right
  C : PMIOPort  Port=5  Side=Left
  c : PMIOPort  Port=6  Side=Right
  wires:
  Three-Phase V-I Measurement/1 -> AC Time Overcurrent Relay2/1(I)  "Iabc"
  AC Time Overcurrent Relay2/2(OT) -> Display/1
  AC Time Overcurrent Relay2/1(C.B) -> Three-Phase Breaker/1  "Relay C"
  connections:
  Three-Phase Breaker/RConn2 -- Three-Phase V-I Measurement/LConn2
  Three-Phase V-I Measurement/RConn2 -- b/RConn1
  Three-Phase V-I Measurement/LConn1 -- Three-Phase Breaker/RConn1
  Three-Phase Breaker/LConn2 -- B/RConn1
  Three-Phase V-I Measurement/RConn1 -- a/RConn1
  Three-Phase Breaker/RConn3 -- Three-Phase V-I Measurement/LConn3
  Three-Phase Breaker/LConn3 -- C/RConn1
  Three-Phase V-I Measurement/RConn3 -- c/RConn1
  Three-Phase Breaker/LConn1 -- A/RConn1

== system Project_microgrid__2016a/Relay W ==
  AC Time Overcurrent Relay2 : Subsystem  mask(AC Time Overcurrent Relay Block){tcpopup=Definite Minimum Time, k=0, alpha=0.02, B=0, PS=100%, TMS=0.1, TDS=5, CTpri=300, CTsec=5, Freq=60, RMSInit=0}
      mask prompts: tcpopup "Trip Characteristic"; PS "Plug Setting (PS) / Low-set (I >)"; TMS "Time Multiplier Setting (TMS)"; TDS "Time Delay Setting (TDS) in sec"; CTpri "Current Transformer Primary (A)"; CTsec "Current Transformer Secondary (A)"; Freq "Fundamental frequency (Hz):"; RMSInit "Initial RMS value:"
      mask help:
      | AC Time Overcurrent Relay Block developed by Dr Rodney Tan
      | Version 1.0 (Jun 2016)
      |
      | AC Time Overcurrent Relay (ANSI/IEEE C37.2 device number 51) that operates when the current exceeds a predetermined value.
      |
      | This relay operates with either a Definite Minimum Time (DMT) or Inverse Definite Minimum Time (IDMT) characteristic.
      |
      | This relay support both IEC 60255 Standard and IEEE Standard C37.112-1996 IDMT trip characteristic.
      mask Help:
      | <b><u>Block Setting</u></b>
      | <b>Trip Characteristic</b>
      | Relay operation mode selection of Definite Minimum Time (DMT), IEC 60255 Standard or IEEE Standard C37.112-1996 Inverse Definite Minimum Time (IDMT).
      | 
      | <b>Plug-Setting(PS) / Low-set (I >)</b>
      | Specify relay pick-up current based on current transformer rating ranging from 25% to 200% with 25% step interval.
      | 
      | <b>Time Multiplier Setting (TMS)</b>
      | Specify time delay multiplier ranging from 0.05 to 1.0 for IDMT relay operation. This setting will be disabled DMT relay operation mode.
      | 
      | <b>Plot Curve Button</b>
      | Plot current Inverse Definite Minimum Time trip curve.
      | 
      | <b>Time Delay Setting (TDS)</b>
      | Specify time delay ranging from 0.05sec to 99sec for Definite Minimum Time relay operation. This setting will be disabled in IDMT relay operation mode.
      | 
      | <b>Current Transformer Primary (A)</b>
      | Specify current transformer primary in Ampere.
      | 
      | <b>Current Transformer Secondary (A)</b>
      | Specify current transformer secondary in Ampere.
      | 
      | <b>Fundamental Frequency (Hz)</b>
      | Specify the RMS current measurement fundamental frequency, in hertz, of the input signal.
      | 
      | <b>Initial RMS Value</b>
      | Specify the RMS current measurement initial RMS value of the output signal.
      | 
      | <b><u>Block Input Output</u></b>
      | <b>I</b>
      | Current input to the AC time overcurrent relay
      | 
      | <b>trip</b>
      | Trip control signal output (1-0), commonly connected to circuit breaker
      | 
      | <b>OT</b>
      | Relay operating time output
      mask TypeOptions tcpopup: Definite Minimum Time | IEC Standard Inverse | IEC Very Inverse | IEC Long Time Inverse | IEC Extremely Inverse | IEC Ultra Inverse | IEEE Moderately Inverse | IEEE Very Inverse | IEEE Extremely Inverse
      mask Callback tcpopup:
      | switch(get_param(gcb,'tcpopup'))
      |     case 'IEC Standard Inverse'
      |         set_param(gcb,'k','0.14');
      |         set_param(gcb,'alpha','0.02');
      |         set_param(gcb,'B','0');
      |         set_param(gcb,'MaskEnables',{'on','off','off','off',...
      |                   'on','on','off','on','on','on','on'});
      |     case 'IEC Very Inverse'
      |         set_param(gcb,'k','13.5');
      |         set_param(gcb,'alpha','1');
      |         set_param(gcb,'B','0');
      |         set_param(gcb,'MaskEnables',{'on','off','off','off',...
      |                   'on','on','off','on','on','on','on'});
      |     case 'IEC Long Time Inverse'
      |         set_param(gcb,'k','120');
      |         set_param(gcb,'alpha','1');
      |         set_param(gcb,'B','0');
      |         set_param(gcb,'MaskEnables',{'on','off','off','off',...
      |                   'on','on','off','on','on','on','on'});
      |     case 'IEC Extremely Inverse'
      |         set_param(gcb,'k','80');
      |         set_param(gcb,'alpha','2');
      |         set_param(gcb,'B','0');
      |         set_param(gcb,'MaskEnables',{'on','off','off','off',...
      |                   'on','on','off','on','on','on','on'});
      |     case 'IEC Ultra Inverse'
      |         set_param(gcb,'k','315.2');
      |         set_param(gcb,'alpha','2.5');
      |         set_param(gcb,'B','0');
      |         set_param(gcb,'MaskEnables',{'on','off','off','off',...
      |                   'on','on','off','on','on','on','on'});
      |     case 'IEEE Moderately Inverse'
      |         set_param(gcb,'k','0.0515');
      |         set_param(gcb,'alpha','0.02');
      |         set_param(gcb,'B','0.114');
      |         set_param(gcb,'MaskEnables',{'on','off','off','off',...
      |                   'on','on','off','on','on','on','on'});
      |     case 'IEEE Very Inverse'
      |         set_param(gcb,'k','19.61');
      |         set_param(gcb,'alpha','2');
      |         set_param(gcb,'B','0.491');
      |         set_param(gcb,'MaskEnables',{'on','off','off','off',...
      |                   'on','on','off','on','on','on','on'});
      |     case 'IEEE Extremely Inverse'
      |         set_param(gcb,'k','28.2');
      |         set_param(gcb,'alpha','2');
      |         set_param(gcb,'B','0.1217');
      |         set_param(gcb,'MaskEnables',{'on','off','off','off',...
      |                   'on','on','off','on','on','on','on'});
      |     otherwise
      |         set_param(gcb,'k','0');
      |         set_param(gcb,'MaskEnables',{'on','off','off','off',...
      |                   'on','off','on','on','on','on','on'});
      | end
      mask TypeOptions PS: 25% | 50% | 75% | 100% | 125% | 150% | 175% | 200%
      mask TypeOptions TMS: 0.05 | 0.1 | 0.15 | 0.2 | 0.25 | 0.3 | 0.35 | 0.4 | 0.45 | 0.5 | 0.55 | 0.6 | 0.65 | 0.7 | 0.75 | 0.8 | 0.85 | 0.9 | 0.95 | 1.0
      mask Callback TDS:
      | TDS = str2double(get_param(gcb,'TDS'));
      | if (TDS > 99)||(TDS < 0.05)||isnan(TDS)
      |     msgbox('TDS must be in the range of 0.05-99 sec',...
      |     'Invalid Value !','error');
      |     set_param(gcb,'TDS','0.1');
      | end
      mask TypeOptions Freq: Irms/Freq
      mask TypeOptions RMSInit: Irms/RMSInit
      mask DialogControl plotbutton Prompt: Plot Curve
      mask DialogControl plotbutton Callback:
      | % Plotting IDMT Curve
      | TMS = str2num(get_param(gcb,'TMS'));
      | k = str2num(get_param(gcb,'k'));
      | alpha = str2num(get_param(gcb,'alpha'));
      | B = str2num(get_param(gcb,'B'));
      | I = 1:20;
      | td = ((k./((I.^alpha)-1))+B)*TMS;
      | loglog(td);
      | set(gcf, 'Position', [200 150 300 500]);
      | switch(get_param(gcb,'tcpopup'))
      |     case 'IEC Standard Inverse'
      |         title('IEC Standard Inverse');
      |         set(gca, 'YTick', (1:10));
      |         ylim([0.1 10]);
      |     case 'IEC Very Inverse'
      |         title('IEC Very Inverse');
      |         set(gca, 'YTick', (1:2:15));
      |         ylim([0.01 15]);
      |     case 'IEC Long Time Inverse'
      |         title('IEC Long Time Inverse');
      |         set(gca, 'YTick', (0:20:120));
      |         ylim([0.1 120]);
      |     case 'IEC Extremely Inverse'
      |         title('IEC Extremely Inverse');
      |         set(gca, 'YTick', (0:5:30));
      |         ylim([0.01 30]);
      |     case 'IEC Ultra Inverse'
      |         title('IEC Ultra Inverse');
      |         set(gca, 'YTick', (0:20:100));
      |         ylim([0.01 100]);
      |     case 'IEEE Moderately Inverse'
      |         title('IEEE Moderately Inverse');
      |         set(gca, 'YTick', (1:5));
      |         ylim([0.01 5]);
      |     case 'IEEE Very Inverse'
      |         title('IEEE Very Inverse');
      |         set(gca, 'YTick', (1:10));
      |         ylim([0.01 10]);
      |     case 'IEEE Extremely Inverse'
      |         title('IEEE Extremely Inverse');
      |         set(gca, 'YTick', (1:10));
      |         ylim([0.01 10]);
      | end
      | 
      | set(gca, 'XTick', [1:10 20]);
      | xlim([1 30]);
      | xlabel('Current (Multiples of Plug Setting)');
      | ylabel('Operating Time (sec)');
      | grid on;
      mask DialogControl RMS Prompt: RMS Current Measurement
      mask Display:
      | disp('(51)');
      | port_label('input', 1, 'I');
      | port_label('output', 1, 'trip');
      | port_label('output', 2, 'OT');
  Display : Display
  Three-Phase V-I Measurement : powerlib/Measurements/Three-Phase V-I Measurement  VoltageMeasurement=no  SetLabelV=off  LabelV=Vabc  Vpu=off  VpuLL=off  CurrentMeasurement=yes  SetLabelI=off  LabelI=Iabc  Ipu=off  Pbase=100e6  Vbase=500e3  OutputType=Complex  PhasorSimulation=off  PSBequivalent=0
  Three-Phase Breaker : powerlib/Elements/Three-Phase Breaker  InitialState=closed  SwitchA=on  SwitchB=on  SwitchC=on  SwitchTimes="[1/60  5/60]"  External=on  BreakerResistance=0.001  SnubberResistance=1e6  SnubberCapacitance=inf  Measurements=None
  A : PMIOPort  Side=Left
  a : PMIOPort  Port=2  Side=Right
  B : PMIOPort  Port=3  Side=Left
  b : PMIOPort  Port=4  Side=Right
  C : PMIOPort  Port=5  Side=Left
  c : PMIOPort  Port=6  Side=Right
  wires:
  Three-Phase V-I Measurement/1 -> AC Time Overcurrent Relay2/1(I)  "Iabc"
  AC Time Overcurrent Relay2/2(OT) -> Display/1
  AC Time Overcurrent Relay2/1(C.B) -> Three-Phase Breaker/1  "Relay C"
  connections:
  Three-Phase Breaker/RConn2 -- Three-Phase V-I Measurement/LConn2
  Three-Phase V-I Measurement/RConn2 -- b/RConn1
  Three-Phase V-I Measurement/LConn1 -- Three-Phase Breaker/RConn1
  Three-Phase Breaker/LConn2 -- B/RConn1
  Three-Phase V-I Measurement/RConn1 -- a/RConn1
  Three-Phase Breaker/RConn3 -- Three-Phase V-I Measurement/LConn3
  Three-Phase Breaker/LConn3 -- C/RConn1
  Three-Phase V-I Measurement/RConn3 -- c/RConn1
  Three-Phase Breaker/LConn1 -- A/RConn1
